simulink library "Library_1"  (R2024a)
settings: Solver=VariableStepAuto  StartTime=0.0  StopTime=10.0  RelTol=1e-3
undefined symbols (not defined in the file): gamma, k, k0
settings Model: Creator=marmr  LastModifiedBy=marmr

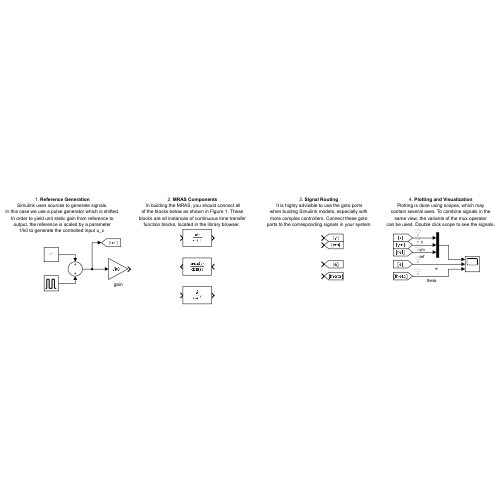
[thumbnail: Simulink's stored preview of the top-level diagram]
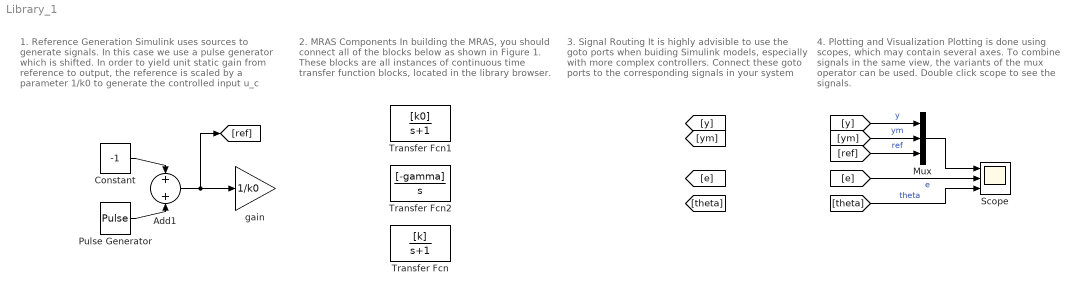
== system Library_1 ==
  note: 4. Plotting and Visualization
      | Plotting is done using scopes, which may
      | contain several axes. To combine signals in the
      | same view, the variants of the mux operator
      | can be used. Double click scope to see the signals.
  note: 2. MRAS Components
      | In building the MRAS, you should connect all
      | of the blocks below as shown in Figure 1. These
      | blocks are all instances of continuous time transfer
      | function blocks, located in the library browser.
  note: 1. Reference Generation
      | Simulink uses sources to generate signals.
      | In this case we use a pulse generator which is shifted.
      | In order to yield unit static gain from reference to
      | output, the reference is scaled by a parameter
      | 1/k0 to generate the controlled input u_c
  note: 3. Signal Routing
      | It is highly advisible to use the goto ports
      | when buiding Simulink models, especially with
      | more complex controllers. Connect these goto
      | ports to the corresponding signals in your system
  Add1 : Sum
  Constant : Constant  Value=-1  SampleTime=0.1
  Mux : Mux  Inputs=3
  Pulse Generator : DiscretePulseGenerator  PulseType=Time based  Amplitude=2  Period=10  PulseWidth=50
  Scope : Scope  NumInputPorts=3
  Transfer Fcn : TransferFcn  Numerator=[k]  Denominator=[1 1]
  Transfer Fcn1 : TransferFcn  Numerator=[k0]  Denominator=[1 1]
  Transfer Fcn2 : TransferFcn  Numerator=[-gamma]  Denominator=[1 0]
  gain : Gain  Gain=1/k0
  wires:
  [theta] -> Scope/3  "theta"
  [ref] -> Mux/3  "ref"
  Pulse Generator/1 -> Add1/2
  Constant/1 -> Add1/1
  [e] -> Scope/2  "e"
  Add1/1 -> gain/1, [ref]
  [ym] -> Mux/2  "ym"
  Mux/1 -> Scope/1
  [y] -> Mux/1  "y"
